simulink model "L_brushless_complessivo"  (R2023b)
settings: Solver=VariableStepAuto  StartTime=0.0  StopTime=3  RelTol=1e-3
libraries: fl_lib x23, fl_ps_legacy_lib x15, nesl_utility x7, ee_lib x1
settings Model: Creator=simon  LastModifiedBy=simon

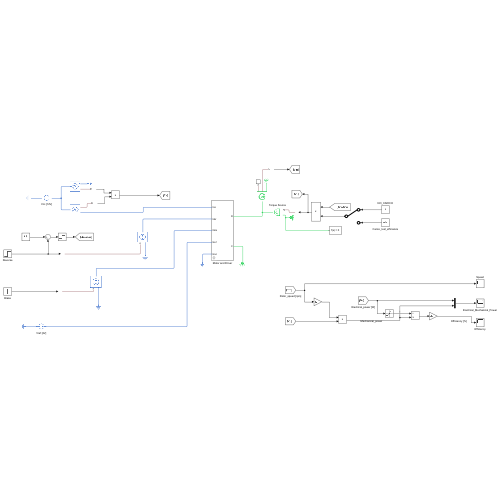
[thumbnail: Simulink's stored preview of the top-level diagram]
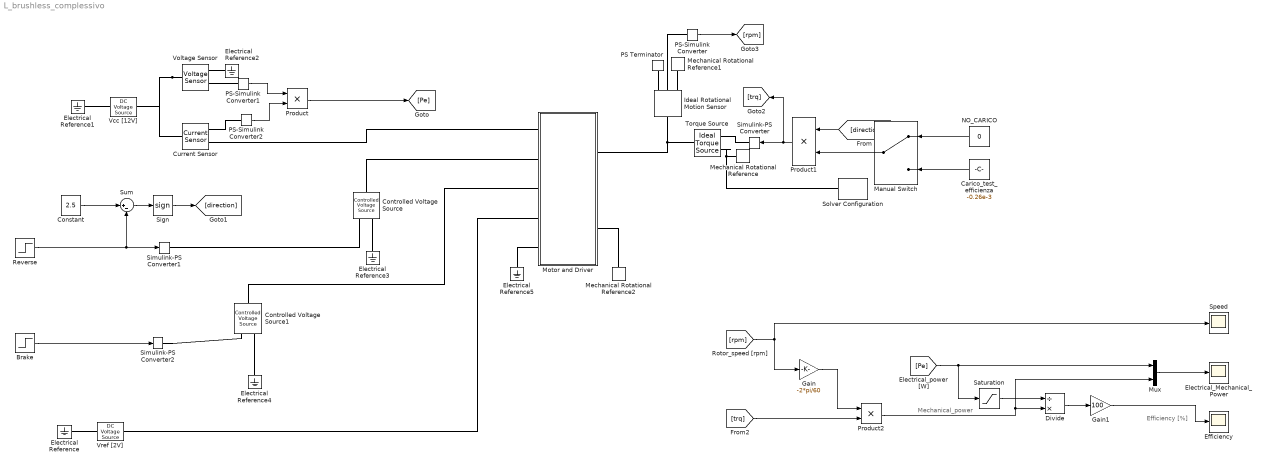
== system L_brushless_complessivo ==
  note: Efficiency [%]
  note: Mechanical_power
  Brake : Step  Time=2  After=5  SampleTime=0
  Carico_test_efficienza : Constant  Value=-0.26e-3
  Constant : Constant  Value=2.5
  Controlled Voltage Source : fl_lib/Electrical/Electrical Sources/Controlled Voltage Source
  Controlled Voltage Source1 : fl_lib/Electrical/Electrical Sources/Controlled Voltage Source
  Current Sensor : fl_lib/Electrical/Electrical Sensors/Current Sensor
  Divide : Product  Inputs=/*
  Efficiency : Scope
  Electrical Reference{,1..5} (6 alike) : fl_lib/Electrical/Electrical Elements/Electrical Reference
  Electrical_Mechanical_Power : Scope
  Gain : Gain  Gain=-2*pi/60
  Gain1 : Gain  Gain=100
  Ideal Rotational Motion Sensor : fl_lib/Mechanical/Mechanical Sensors/Ideal Rotational Motion Sensor  reference=foundation.enum.MeasurementReference.difference  acceleration_port=false  velocity_port=true  position_port=true  wrap_angle=false  offset=0 rad
  Manual Switch : ManualSwitch
  Mechanical Rotational Reference : fl_lib/Mechanical/Rotational Elements/Mechanical Rotational Reference
  Mechanical Rotational Reference1 : fl_lib/Mechanical/Rotational Elements/Mechanical Rotational Reference
  Mechanical Rotational Reference2 : fl_lib/Mechanical/Rotational Elements/Mechanical Rotational Reference
  Motor and Driver : Subsystem  Tag=PublishSubsystem  mask(Servomotor & Driver){Vcc=12, I0=44e-3, T_i=0.5e-3, eta=41, rpm_eta=40000, trq_eta=0.26e-3, trq_stall=0.44e-3, Kp=0.0000001, Ki=0.000004, Vref_max=5, rpm_max=100000, J=5e-10, rpm0=0}
      mask prompts: Vcc "Nominal voltage (V)"; I0 "No-load DC current to driver (A)"; T_i "Current loop time constant (s)"; eta "Efficiency (%)"; rpm_eta "Speed at which efficiency measured (rpm)"; trq_eta "Torque at which efficiency measured  (Nm)"; trq_stall "Stall torque (Nm)"; Kp "Proportional gain"; Ki "Integral gain"; Vref_max "Maximum reference voltage (V)"; rpm_max "Speed at maximum reference voltage (rpm)"; J "Rotor inerita (kg*m^2)"; rpm0 "Rotor initial speed (rpm)"
      mask help: Implements an abstracted model of a servomotor and driver configured for closed-loop speed control.
      mask DialogControl ParameterTabVar0 Prompt: Electrical
      mask DialogControl ParameterTabVar01 Prompt: Efficiency
      mask DialogControl ParameterTabVar012 Prompt: Mechanical
      mask DialogControl ParameterTabVar0123 Prompt: Controller
  Mux : Mux  Inputs=2
  NO_CARICO : Constant  Value=0
  PS Terminator : fl_lib/Physical Signals/Sinks/PS Terminator
  PS-Simulink Converter : nesl_utility/PS-Simulink Converter  PhysicalDomain=network_engine_domain  SubClassName=ps_output  LeftPortType=input  RightPortType=output  PseudoPeriodic=off  Frequencies=[]  VectorFormat=inherit  Unit=inherit  AffineConversion=off
  PS-Simulink Converter1 : nesl_utility/PS-Simulink Converter  PhysicalDomain=network_engine_domain  SubClassName=ps_output  LeftPortType=input  RightPortType=output  PseudoPeriodic=off  Frequencies=[]  VectorFormat=inherit  Unit=inherit  AffineConversion=off
  PS-Simulink Converter2 : nesl_utility/PS-Simulink Converter  PhysicalDomain=network_engine_domain  SubClassName=ps_output  LeftPortType=input  RightPortType=output  PseudoPeriodic=off  Frequencies=[]  VectorFormat=inherit  Unit=inherit  AffineConversion=off
  Product : Product
  Product1 : Product
  Product2 : Product
  Reverse : Step  After=5  SampleTime=0
  Saturation : Saturate  UpperLimit=inf  LowerLimit=1e-3
  Sign : Signum
  Simulink-PS Converter : nesl_utility/Simulink-PS Converter  PhysicalDomain=network_engine_domain  SubClassName=ps_input  LeftPortType=input  RightPortType=output  PseudoPeriodic=off  Frequencies=[]  NoiseDistribution=none  NoiseParameters=[]  Unit=1  AffineConversion=off  FilteringAndDerivatives=provide  SimscapeFilterOrder=1  InputFilterTimeConstant=0.001  UdotUserProvided=0
  Simulink-PS Converter1 : nesl_utility/Simulink-PS Converter  PhysicalDomain=network_engine_domain  SubClassName=ps_input  LeftPortType=input  RightPortType=output  PseudoPeriodic=off  Frequencies=[]  NoiseDistribution=none  NoiseParameters=[]  Unit=1  AffineConversion=off  FilteringAndDerivatives=provide  SimscapeFilterOrder=1  InputFilterTimeConstant=0.001  UdotUserProvided=0
  Simulink-PS Converter2 : nesl_utility/Simulink-PS Converter  PhysicalDomain=network_engine_domain  SubClassName=ps_input  LeftPortType=input  RightPortType=output  PseudoPeriodic=off  Frequencies=[]  NoiseDistribution=none  NoiseParameters=[]  Unit=1  AffineConversion=off  FilteringAndDerivatives=provide  SimscapeFilterOrder=1  InputFilterTimeConstant=0.001  UdotUserProvided=0
  Solver Configuration : nesl_utility/Solver Configuration  PhysicalDomain=network_engine_domain  SubClassName=solver  LeftPortType=input  RightPortType=generic  Tones=[]  Harmonics=[]  SimulateNoise=off  Profile=off  UseLocalSampling=off  EnableSwitchedLinearOptims=on  FrequencyDomain=off  UseCCode=off  RelTol=0.001  AbsTol=0.001  MinStep=1e-09  ToWorkspace=off  RevertToSquareIcSolve=off  NumHomotopyIterations=100  PhasorMode=off  PhasorModeNumHarmonics=1  ConsistencySolver=NEWTON_XTOL_AFTER_FTOL  IndexReductionMethod=DerivativeReplacement  DoDC=off  ResidualTolerance=1e-09  ConsistencyTolSource=LOCAL  ConsistencyAbsTol=0.001  ConsistencyRelTol=0.001  ConsistencyTolFactor=1e-9  UseLocalSolver=off  LocalSolverChoice=NE_BACKWARD_EULER_ADVANCER  ResolveIndetEquations=on  FunctionEvalNumThread=1  LocalSolverSampleTime=0.001  DoFixedCost=off  MaxNonlinIter=3  MaxModeIter=2  ComputeImpulses=off  ImpulseIterations=2  LinearAlgebra=auto  LinearAlgebraNumThread=0  EquationFormulation=NE_TIME_EF  DelaysMemoryBudget=1024  AutomaticFiltering=on  FilteringTimeConstant=0.001  PartitionStorageMethod=AS_NEEDED  PartitionMemoryBudget=1024  PartitionMethod=ROBUST  MultibodyUseLocalSolver=off  MultibodyLocalSolverChoice=ODE1  MultibodyLocalSolverSampleTime=0.001
  Speed : Scope
  Sum : Sum  Inputs=|+-
  Torque Source : fl_lib/Mechanical/Mechanical Sources/Ideal Torque Source
  Vcc [12V] : fl_lib/Electrical/Electrical Sources/DC Voltage Source  v0=12 V
  Voltage Sensor : fl_lib/Electrical/Electrical Sensors/Voltage Sensor
  Vref [2V] : fl_lib/Electrical/Electrical Sources/DC Voltage Source  v0=2 V
  wires:
  Reverse/1 -> Sum/2, Simulink-PS Converter1/1
  PS-Simulink Converter2/1 -> Product/2
  PS-Simulink Converter1/1 -> Product/1
  Brake/1 -> Simulink-PS Converter2/1
  Product/1 -> [Pe]
  Sign/1 -> [direction]
  Sum/1 -> Sign/1
  Constant/1 -> Sum/1
  Carico_test_efficienza/1 -> Manual Switch/2
  Product1/1 -> [trq], Simulink-PS Converter/1
  PS-Simulink Converter/1 -> [rpm]
  [direction] -> Product1/1
  NO_CARICO/1 -> Manual Switch/1
  Manual Switch/1 -> Product1/2
  Gain1/1 -> Efficiency/1
  Mux/1 -> Electrical_Mechanical_Power/1
  Divide/1 -> Gain1/1
  [trq] -> Product2/2
  [Pe] -> Saturation/1, Mux/1
  [rpm] -> Speed/1, Gain/1
  Product2/1 -> Mux/2, Divide/2
  Saturation/1 -> Divide/1
  Gain/1 -> Product2/1
  connections:
  Voltage Sensor/LConn1 -- Vcc [12V]/LConn1 -- Current Sensor/LConn1
  Electrical Reference4/LConn1 -- Controlled Voltage Source1/RConn2
  Voltage Sensor/RConn1 -- PS-Simulink Converter1/LConn1
  Simulink-PS Converter2/RConn1 -- Controlled Voltage Source1/RConn1
  Electrical Reference1/LConn1 -- Vcc [12V]/RConn1
  Current Sensor/RConn1 -- PS-Simulink Converter2/LConn1
  Electrical Reference/LConn1 -- Vref [2V]/RConn1
  Controlled Voltage Source1/LConn1 -- Motor and Driver/LConn3
  Controlled Voltage Source/RConn2 -- Electrical Reference3/LConn1
  Simulink-PS Converter1/RConn1 -- Controlled Voltage Source/RConn1
  Electrical Reference2/LConn1 -- Voltage Sensor/RConn2
  Controlled Voltage Source/LConn1 -- Motor and Driver/LConn2
  Current Sensor/RConn2 -- Motor and Driver/LConn1
  Vref [2V]/LConn1 -- Motor and Driver/LConn4
  Electrical Reference5/LConn1 -- Motor and Driver/LConn5
  Motor and Driver/RConn2 -- Mechanical Rotational Reference2/LConn1
  Mechanical Rotational Reference/LConn1 -- Torque Source/RConn2 -- Solver Configuration/RConn1
  Torque Source/LConn1 -- Motor and Driver/RConn1 -- Ideal Rotational Motion Sensor/LConn1
  Torque Source/RConn1 -- Simulink-PS Converter/RConn1
  PS Terminator/LConn1 -- Ideal Rotational Motion Sensor/RConn3
  Mechanical Rotational Reference1/LConn1 -- Ideal Rotational Motion Sensor/RConn1
  Ideal Rotational Motion Sensor/RConn2 -- PS-Simulink Converter/LConn1

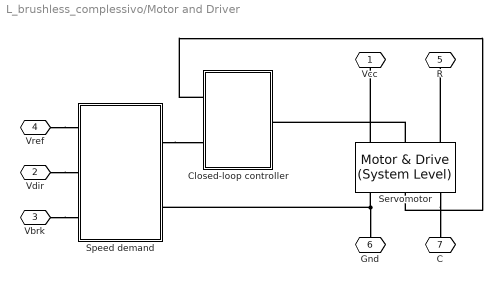
== system L_brushless_complessivo/Motor and Driver ==
  Closed-loop controller : Subsystem
  Servomotor : ee_lib/Electromechanical/Motor & Drive (System Level)  torque_speed_param=1  overtorque_param=ee.enum.electromech.overtorque.no  T_t="[  trq_stall trq_stall trq_stall  0 ] N*m"  T_t_intermittent=[.36, .32, .28, 0] N*m  T_t_2D=[.09, .09, .09; .08, .08, .08; .07, .07, .07; 0, 0, 0] N*m  T_t_intermittent_2D=[.36, .36, .36; .32, .32, .32; .28, .28, .28; 0, 0, 0] N*m  w_t="[  0 rpm_max 2*rpm_max 2.1*rpm_max ] rpm"  vdc_t=[6, 12, 24] V  torque_max=0.1 N*m  power_max=30 W  torque_max_intermittent=0.4 N*m  power_max_intermittent=120 W  time_overtorque=30 s  time_recover=60 s  Tc=T_i s  EnableSwitch=simscape.enum.onoff.off  losses_param=1  eff=eta  w_eff=rpm_eta rpm  T_eff=trq_eta N*m  Piron=0 W  Pbase=Vcc*I0 W  w_eff_vec=[-8000 -4000 0 4000 8000] rpm  T_eff_vec=[0 0.03 0.06 0.09] N*m  v_eff_vec=[100, 250, 400] V  losses_mat=[1.49 1.67 2.21 3.10; 0.42 0.69 1.14 2.03; 0.06 0.24 0.78 1.68; 0.42 0.69 1.14 2.03; 1.49 1.67 2.21 3.10] W  efficiency_mat=[95 95 95 95; 95 95 95 95; 95 95 95 95; 95 95 95 95; 95 95 95 95]  losses_mat_3D=ones(5, 4, 3) W  efficiency_mat_3D=95 * ones(5, 4, 3)  Res=0 Ohm  enable_fault=simscape.enum.onoff.off  fault_condition=1  fault_threshold=0.5  J=J kg*m^2  lam=0 N*m/(rad/s)  speed0=rpm0 rpm  faulted_specify=off  faulted_priority=None  faulted=0  faulted_nominal_specify=off  faulted_nominal_unit=1  faulted_nominal_value=1  isSwitchedOff_specify=off  isSwitchedOff_priority=None  isSwitchedOff=0  isSwitchedOff_nominal_specify=off  isSwitchedOff_nominal_unit=1  isSwitchedOff_nominal_value=1  torqueLimitContinuous_specify=off  torqueLimitContinuous_priority=None  torqueLimitContinuous=0 N*m  torqueLimitContinuous_nominal_specify=off  torqueLimitContinuous_nominal_unit=N*m  torqueLimitContinuous_nominal_value=1  alpha=3.93e-3 1/K  Tmeas=25 degC  Tmeas2=125 degC  losses_mat_T2=[1.49, 1.74, 2.49, 3.74; .42, .67, 1.42, 2.67; .06, .31, 1.06, 2.31; .42, .67, 1.42, 2.67; 1.49, 1.74, 2.49, 3.74] W  efficiency_mat_T2=[95, 95, 95, 95; 95, 95, 95, 95; 95, 95, 95, 95; 95, 95, 95, 95; 95, 95, 95, 95]  losses_mat_3D_T2=ones(5, 4, 3) W  efficiency_mat_3D_T2=95 * ones(5, 4, 3)  thermal_mass=100 J/K  initial_temperature=25 degC
  Speed demand : Subsystem
  Vcc : PMIOPort  Side=Left
  Vdir : PMIOPort  Port=2  Side=Left
  Vbrk : PMIOPort  Port=3  Side=Left
  Vref : PMIOPort  Port=4  Side=Left
  R : PMIOPort  Port=5  Side=Right
  Gnd : PMIOPort  Port=6  Side=Left
  C : PMIOPort  Port=7  Side=Right
  connections:
  Servomotor/LConn2 -- Closed-loop controller/RConn1
  Servomotor/RConn3 -- C/RConn1
  Servomotor/RConn1 -- Gnd/RConn1 -- Speed demand/RConn2
  Vbrk/RConn1 -- Speed demand/LConn3
  Vdir/RConn1 -- Speed demand/LConn2
  Vref/RConn1 -- Speed demand/LConn1
  Servomotor/LConn3 -- R/RConn1
  Servomotor/LConn1 -- Vcc/RConn1
  Closed-loop controller/LConn1 -- Servomotor/RConn2
  Speed demand/RConn1 -- Closed-loop controller/LConn2

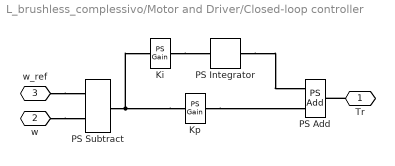
== system L_brushless_complessivo/Motor and Driver/Closed-loop controller ==
  Ki : fl_ps_legacy_lib/Legacy Physical Signals/Functions/PS Gain  gain=Ki
  Kp : fl_ps_legacy_lib/Legacy Physical Signals/Functions/PS Gain  gain=Kp
  PS Add : fl_ps_legacy_lib/Legacy Physical Signals/Functions/PS Add
      settings: InternalSimscapePortConfiguration="{\"Bottom\":[],\"Left\":[{\"id\":\"I1\",\"label\":\"\",\"type\":\"input\"},{\"id\":\"I2\",\"label\":\"\",\"type\":\"input\"}],\"Right\":[{\"id\":\"O\",\"label\":\"\",\"type\":\"output\"}],\"Top\":[]}"
  PS Integrator : fl_ps_legacy_lib/Legacy Physical Signals/Linear Operators/PS Integrator  x0=0
      settings: InternalSimscapePortConfiguration="{\"Bottom\":[],\"Left\":[{\"id\":\"I\",\"label\":\"\",\"type\":\"input\"}],\"Right\":[{\"id\":\"O\",\"label\":\"\",\"type\":\"output\"}],\"Top\":[]}"
  PS Subtract : fl_ps_legacy_lib/Legacy Physical Signals/Functions/PS Subtract
  Tr : PMIOPort  Side=Right
  w : PMIOPort  Port=2  Side=Left
  w_ref : PMIOPort  Port=3  Side=Left
  connections:
  w/RConn1 -- PS Subtract/LConn2
  w_ref/RConn1 -- PS Subtract/LConn1
  Tr/RConn1 -- PS Add/RConn1
  PS Integrator/RConn1 -- PS Add/LConn1
  Kp/RConn1 -- PS Add/LConn2
  Ki/RConn1 -- PS Integrator/LConn1
  Kp/LConn1 -- PS Subtract/RConn1 -- Ki/LConn1

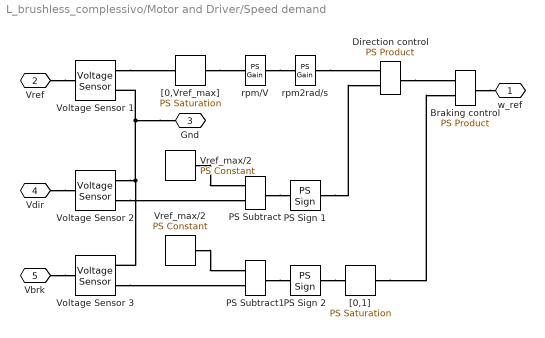
== system L_brushless_complessivo/Motor and Driver/Speed demand ==
  " Vref_max/2 " : fl_lib/Physical Signals/Sources/PS Constant  constant=Vref_max/2
  Braking control : fl_ps_legacy_lib/Legacy Physical Signals/Functions/PS Product
  Direction control : fl_ps_legacy_lib/Legacy Physical Signals/Functions/PS Product
  PS Sign 1 : fl_ps_legacy_lib/Legacy Physical Signals/Nonlinear Operators/PS Sign
      settings: InternalSimscapePortConfiguration="{\"Bottom\":[],\"Left\":[{\"id\":\"I\",\"label\":\"\",\"type\":\"input\"}],\"Right\":[{\"id\":\"O\",\"label\":\"\",\"type\":\"output\"}],\"Top\":[]}"
  PS Sign 2 : fl_ps_legacy_lib/Legacy Physical Signals/Nonlinear Operators/PS Sign
      settings: InternalSimscapePortConfiguration="{\"Bottom\":[],\"Left\":[{\"id\":\"I\",\"label\":\"\",\"type\":\"input\"}],\"Right\":[{\"id\":\"O\",\"label\":\"\",\"type\":\"output\"}],\"Top\":[]}"
  PS Subtract : fl_ps_legacy_lib/Legacy Physical Signals/Functions/PS Subtract
  PS Subtract1 : fl_ps_legacy_lib/Legacy Physical Signals/Functions/PS Subtract
  Voltage Sensor 1 : fl_lib/Electrical/Electrical Sensors/Voltage Sensor
  Voltage Sensor 2 : fl_lib/Electrical/Electrical Sensors/Voltage Sensor
  Voltage Sensor 3 : fl_lib/Electrical/Electrical Sensors/Voltage Sensor
  Vref_max/2 : fl_lib/Physical Signals/Sources/PS Constant  constant=Vref_max/2
  "[0,1]" : fl_ps_legacy_lib/Legacy Physical Signals/Nonlinear Operators/PS Saturation  upper_limit=5  lower_limit=0
      settings: InternalSimscapePortConfiguration="{\"Bottom\":[],\"Left\":[{\"id\":\"I\",\"label\":\"\",\"type\":\"input\"}],\"Right\":[{\"id\":\"O\",\"label\":\"\",\"type\":\"output\"}],\"Top\":[]}"
  "[0,Vref_max]" : fl_ps_legacy_lib/Legacy Physical Signals/Nonlinear Operators/PS Saturation  upper_limit=Vref_max  lower_limit=0
      settings: InternalSimscapePortConfiguration="{\"Bottom\":[],\"Left\":[{\"id\":\"I\",\"label\":\"\",\"type\":\"input\"}],\"Right\":[{\"id\":\"O\",\"label\":\"\",\"type\":\"output\"}],\"Top\":[]}"
  rpm/V : fl_ps_legacy_lib/Legacy Physical Signals/Functions/PS Gain  gain=rpm_max/Vref_max
  rpm2rad/s : fl_ps_legacy_lib/Legacy Physical Signals/Functions/PS Gain  gain=2*pi/60
  w_ref : PMIOPort  Side=Right
  Vref : PMIOPort  Port=2  Side=Left
  Gnd : PMIOPort  Port=3  Side=Right
  Vdir : PMIOPort  Port=4  Side=Left
  Vbrk : PMIOPort  Port=5  Side=Left
  connections:
  "[0,1]"/RConn1 -- Braking control/LConn2
  Braking control/RConn1 -- w_ref/RConn1
  Direction control/RConn1 -- Braking control/LConn1
  PS Sign 2/RConn1 -- "[0,1]"/LConn1
  PS Subtract1/RConn1 -- PS Sign 2/LConn1
  " Vref_max/2 "/RConn1 -- PS Subtract1/LConn1
  Voltage Sensor 3/RConn1 -- PS Subtract1/LConn2
  Vbrk/RConn1 -- Voltage Sensor 3/LConn1
  Vref_max/2/RConn1 -- PS Subtract/LConn1
  Voltage Sensor 2/RConn1 -- PS Subtract/LConn2
  PS Sign 1/RConn1 -- Direction control/LConn2
  rpm2rad/s/RConn1 -- Direction control/LConn1
  PS Subtract/RConn1 -- PS Sign 1/LConn1
  Vdir/RConn1 -- Voltage Sensor 2/LConn1
  Gnd/RConn1 -- Voltage Sensor 3/RConn2 -- Voltage Sensor 2/RConn2 -- Voltage Sensor 1/RConn2
  Vref/RConn1 -- Voltage Sensor 1/LConn1
  rpm/V/RConn1 -- rpm2rad/s/LConn1
  "[0,Vref_max]"/RConn1 -- rpm/V/LConn1
  Voltage Sensor 1/RConn1 -- "[0,Vref_max]"/LConn1
